simulink model "scex"  (Simulink 8.5)
settings: Solver=ode45  SolverMode=SingleTasking  StartTime=0.0  StopTime=0.06  RelTol=1e-3  AbsTol=1e-6
libraries: elements x4, inputs x1
settings Model: Creator=PC  LastModifiedBy=PC
settings DataIOCC: LimitDataPoints=off
settings OptimizationCC: BlockReduction=off  BooleanDataType=off  ExpressionDepthLimit=128
settings DebuggingCC: SaveWithParameterizedLinksMsg=none  SignalResolutionControl=TryResolveAllWithWarning  MultiTaskDSMMsg=warning  MultiTaskCondExecSysMsg=none  FcnCallInpInsideContextMsg=EnableAllAsError  StateNameClashWarn=none  StrictBusMsg=None
settings HardwareCC: TargetUnknown=on
settings RTWCC: TemplateMakefile=grt_vc.tmf

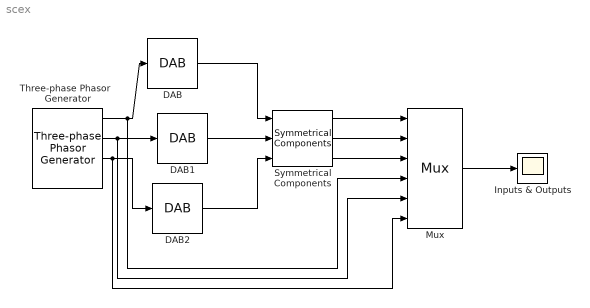
== system scex ==
  DAB : elements/DAB  filter=on  approx=Bessel  order=2  numerator=[]  denominator=[]  freq=180  resdis=on  vertres=12  xmax=1  winsize=40  G=1.0  fs=60*40
  DAB1 : elements/DAB  filter=on  approx=Bessel  order=2  numerator=[]  denominator=[]  freq=180  resdis=on  vertres=12  xmax=1  winsize=40  G=1.0  fs=60*40
  DAB2 : elements/DAB  filter=on  approx=Bessel  order=2  numerator=[]  denominator=[]  freq=180  resdis=on  vertres=12  xmax=1  winsize=40  G=1.0  fs=60*40
  Inputs & Outputs : Scope
      settings: TickLabels=on  YMin=-1  YMax=1
  Mux : Mux  Inputs=6
  Symmetrical Components : elements/Symmetrical Components  ortho_instant=Instantaneous  powerfre=60  samplefre=60*40
  Three-phase Phasor   Generator : inputs/Three-phase Phasor   Generator  phase_type=Phase quantities-symmetrical  phase1=[1 0]  phase2=[0 150]  phase3=[0 -50]  f=60  to=0
  wires:
  DAB2/1 -> Symmetrical Components/3
  DAB/1 -> Symmetrical Components/1
  DAB1/1 -> Symmetrical Components/2
  Three-phase Phasor   Generator/1 -> DAB/1, Mux/4
  Three-phase Phasor   Generator/2 -> DAB1/1, Mux/5
  Three-phase Phasor   Generator/3 -> DAB2/1, Mux/6
  Symmetrical Components/1 -> Mux/1
  Symmetrical Components/2 -> Mux/2
  Symmetrical Components/3 -> Mux/3
  Mux/1 -> Inputs & Outputs/1
